simulink model "koshi"  (R2014a)
settings: Solver=ode45  StartTime=0.0  StopTime=30  RelTol=1e-3
libraries: simulink x2
settings Model: Creator=Alex  LastModifiedBy=Alex

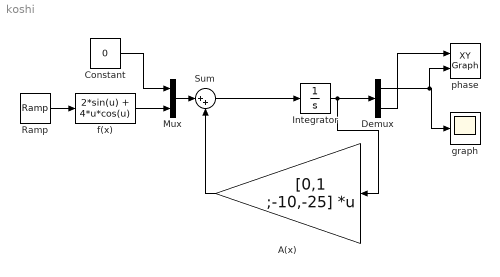
== system koshi ==
  A(x) : Gain  Gain=[0,1 ;-10,-25]  Multiplication=Matrix(K*u) (u vector)
  Constant : Constant  Value=0
  Demux : Demux  Outputs=2
  Integrator : Integrator
  Mux : Mux  Inputs=2
  Ramp : simulink/Sources/Ramp  slope=1  start=0  X0=0
  Sum : Sum  Inputs=|++
  f(x) : Fcn  Expr=2*sin(u) + 4*u*cos(u)
  graph : Scope
  phase : simulink/Sinks/XY Graph  xmin=-5  xmax=5  ymin=-5  ymax=5  st=0.01
  wires:
  f(x)/1 -> Mux/2
  Ramp/1 -> f(x)/1
  Constant/1 -> Mux/1
  Mux/1 -> Sum/1
  Sum/1 -> Integrator/1
  A(x)/1 -> Sum/2
  Integrator/1 -> Demux/1, A(x)/1
  Demux/1 -> phase/2, graph/1
  Demux/2 -> phase/1
